simulink model "cx06_MA"  (Simulink 7.5)
settings: Solver=FixedStepDiscrete  StartTime=0.0  StopTime=10.0  RelTol=1e-3
undefined symbols (not defined in the file or in its folder): DiscIntNeverNeededParam, ECU555, int, motohawk_build_version, motohawk_trunc_name, motohawk_vardec_path
libraries: MotoHawk_lib x811, simulink x43, simulink_need_slupdate x1
(part 7 of 10)

== system cx06_MA/Strategy/Hybrid Control Code/Activation of Traction Control ==
  Inputs : Inport  OutDataType=sfix(16)  OutScaling=2^0
  Data1 : DataTypeConversion  OutDataTypeMode=uint8  OutDataType=sfix(16)  OutScaling=2^0  OutDataTypeStr=uint8
  Data2 : DataTypeConversion  OutDataTypeMode=uint8  OutDataType=sfix(16)  OutScaling=2^0  OutDataTypeStr=uint8
  Logical Operator : Logic  Operator=NOT  AllPortsSameDT=off  OutDataTypeMode=boolean  OutDataTypeStr=boolean
  Logical Operator1 : Logic  AllPortsSameDT=off  OutDataTypeMode=boolean  OutDataTypeStr=boolean
  Logical Operator2 : Logic  Operator=OR  AllPortsSameDT=off  OutDataTypeMode=boolean  OutDataTypeStr=boolean
  Logical Operator3 : Logic  Operator=OR  AllPortsSameDT=off  OutDataTypeMode=boolean  OutDataTypeStr=boolean
  Logical Operator4 : Logic  AllPortsSameDT=off  OutDataTypeMode=boolean  OutDataTypeStr=boolean
  Merge : Merge
  Merge1 : Merge  AllowUnequalInputPortWidths=on
  RRef_Wheel Diff : Subsystem  TreatAsAtomicUnit=on
  Switch Case : SwitchCase  CaseConditions={0,1}  ShowDefaultCase=off
  Wheel_Acceleration : Subsystem  TreatAsAtomicUnit=on
  motohawk_calibration : MotoHawk_lib/Calibration & Probing Blocks/motohawk_calibration  nam='Slip_Determine_Mode'  val=1  storage=Calibration  show_more=off  name_source=Use Parameter  data_type=Inherit from 'Default Value'  read_level=1  write_level=1  ovr_cals=on  view_as=Number  enum_struct={'Disabled', 'Enabled'}  vector_style=Wide Row  use_help_units=off  help=''  units=''  use_header_enum=off  row_header_enum={}  col_header_enum={}  use_min_max=off  min_val=-inf  max_val=inf  use_precision=off  precision=''  gain=1  offset=0  exp=1  use_mototune_group=off  mototune_group=motohawk_vardec_path(gcb)
  motohawk_data_def : MotoHawk_lib/Data Storage Blocks/motohawk_data_def  nam='inhibitTC'  container_nam=''  data=1  typ=uint8  struct_nam='MyStruct'  storage=NonVolatile  outputRef=off  use_vardec=on  window=Calibration  read_level=1  write_level=1  ovr_cals=on  view_as=Enumeration  enum_struct={'False','True'}  vector_style=Wide Row  use_help_units=on  help=''  units=''  use_header_enum=off  row_header_enum=''  col_header_enum=''  use_min_max=off  min_val=-inf  max_val=inf  use_precision=off  precision=''  gain=1  offset=0  exp=1  use_mototune_group=off  mototune_group=motohawk_vardec_path(gcb)  eval_name=inhibitTC  data_stores=motohawk_sfun_data_def_data_stores  struct_instances=motohawk_sfun_data_def_struct_instances  vardecs=motohawk_sfun_data_def_vardecs
  motohawk_data_def1 : MotoHawk_lib/Data Storage Blocks/motohawk_data_def  nam='TCVersion'  container_nam=''  data=1  typ=uint8  struct_nam='MyStruct'  storage=NonVolatile  outputRef=off  use_vardec=on  window=Calibration  read_level=1  write_level=1  ovr_cals=on  view_as=Enumeration  enum_struct={'Automatic','Manual'}  vector_style=Wide Row  use_help_units=on  help=''  units=''  use_header_enum=off  row_header_enum=''  col_header_enum=''  use_min_max=off  min_val=-inf  max_val=inf  use_precision=off  precision=''  gain=1  offset=0  exp=1  use_mototune_group=off  mototune_group=motohawk_vardec_path(gcb)  eval_name=TCVersion  data_stores=motohawk_sfun_data_def_data_stores  struct_instances=motohawk_sfun_data_def_struct_instances  vardecs=motohawk_sfun_data_def_vardecs
  motohawk_data_def2 : MotoHawk_lib/Data Storage Blocks/motohawk_data_def  nam='TC_Front_Slip'  container_nam=''  data=0  typ=uint8  struct_nam='MyStruct'  storage=Volatile  outputRef=off  use_vardec=off  window=Calibration  read_level=1  write_level=1  ovr_cals=on  view_as=Number  enum_struct={'Disabled', 'Enabled'}  vector_style=Wide Row  use_help_units=on  help=''  units=''  use_header_enum=off  row_header_enum=''  col_header_enum=''  use_min_max=off  min_val=-inf  max_val=inf  use_precision=off  precision=''  gain=1  offset=0  exp=1  use_mototune_group=off  mototune_group=motohawk_vardec_path(gcb)  eval_name=TC_Front_Slip  data_stores=motohawk_sfun_data_def_data_stores  struct_instances=motohawk_sfun_data_def_struct_instances  vardecs=motohawk_sfun_data_def_vardecs
  motohawk_data_def3 : MotoHawk_lib/Data Storage Blocks/motohawk_data_def  nam='TC_Rear_Slip'  container_nam=''  data=0  typ=uint8  struct_nam='MyStruct'  storage=Volatile  outputRef=off  use_vardec=off  window=Calibration  read_level=1  write_level=1  ovr_cals=on  view_as=Number  enum_struct={'Disabled', 'Enabled'}  vector_style=Wide Row  use_help_units=on  help=''  units=''  use_header_enum=off  row_header_enum=''  col_header_enum=''  use_min_max=off  min_val=-inf  max_val=inf  use_precision=off  precision=''  gain=1  offset=0  exp=1  use_mototune_group=off  mototune_group=motohawk_vardec_path(gcb)  eval_name=TC_Rear_Slip  data_stores=motohawk_sfun_data_def_data_stores  struct_instances=motohawk_sfun_data_def_struct_instances  vardecs=motohawk_sfun_data_def_vardecs
  motohawk_data_read : MotoHawk_lib/Data Storage Blocks/motohawk_data_read  source=Lookup By Name  structure=Scalar  operation=Read scalar from location by index  sz_vec=4  sz_row=2  sz_col=3  typ=uint8  nam='inhibitTC'  checkNull=on  struct_inst_name='Struct1'  struct_nam='MyStruct'
  motohawk_data_read1 : MotoHawk_lib/Data Storage Blocks/motohawk_data_read  source=Lookup By Name  structure=Scalar  operation=Read scalar from location by index  sz_vec=4  sz_row=2  sz_col=3  typ=uint8  nam='TCVersion'  checkNull=on  struct_inst_name='Struct1'  struct_nam='MyStruct'
  motohawk_data_write : MotoHawk_lib/Data Storage Blocks/motohawk_data_write  source=Lookup By Name  structure=Scalar  operation=Write scalar into location by index  sz_vec=-1  sz_row=3  sz_col=2  typ=uint8  nam='TC_Front_Slip'  checkNull=on  write_read_only=off  struct_inst_name='Struct1'  struct_name='MyStruct'
  motohawk_data_write1 : MotoHawk_lib/Data Storage Blocks/motohawk_data_write  source=Lookup By Name  structure=Scalar  operation=Write scalar into location by index  sz_vec=-1  sz_row=3  sz_col=2  typ=uint8  nam='TC_Rear_Slip'  checkNull=on  write_read_only=off  struct_inst_name='Struct1'  struct_name='MyStruct'
  motohawk_probe : MotoHawk_lib/Calibration & Probing Blocks/motohawk_probe  nam='Front_Slip'  show_more=on  name_source=Use Parameter  read_level=1  view_as=Number  enum_struct={'Disabled', 'Enabled'}  vector_style=Wide Row  use_help_units=off  help=''  units=''  use_header_enum=off  row_header_enum={}  col_header_enum={}  use_precision=off  precision=''  gain=1  offset=0  exp=1  use_mototune_group=off  mototune_group=motohawk_vardec_path(gcb)
  motohawk_probe1 : MotoHawk_lib/Calibration & Probing Blocks/motohawk_probe  nam='Rear_Slip'  show_more=on  name_source=Use Parameter  read_level=1  view_as=Number  enum_struct={'Disabled', 'Enabled'}  vector_style=Wide Row  use_help_units=off  help=''  units=''  use_header_enum=off  row_header_enum={}  col_header_enum={}  use_precision=off  precision=''  gain=1  offset=0  exp=1  use_mototune_group=off  mototune_group=motohawk_vardec_path(gcb)
  Front_Slip? : Outport  OutDataType=sfix(16)  OutScaling=2^0
  wires:
  motohawk_data_read/1 -> Logical Operator/1
  Logical Operator/1 -> Logical Operator1/1, Logical Operator4/1
  Logical Operator1/1 -> Front_Slip?/1, Data1/1
  motohawk_data_read1/1 -> Logical Operator3/1, Logical Operator2/1
  Logical Operator2/1 -> motohawk_probe/1, Logical Operator1/2  "Front_Slip?"
  Data1/1 -> motohawk_data_write/1
  Data2/1 -> motohawk_data_write1/1
  Logical Operator4/1 -> Data2/1
  Inputs/1 -> RRef_Wheel Diff/1(Inputs), Wheel_Acceleration/1(Inputs)
  Switch Case/1 -> RRef_Wheel Diff/Action
  Merge/1 -> Logical Operator2/2
  Merge1/1 -> Logical Operator3/2
  RRef_Wheel Diff/1(Front_Slip?) -> Merge/1
  RRef_Wheel Diff/2(Rear_Slip?) -> Merge1/1
  motohawk_calibration/1 -> Switch Case/1
  Switch Case/2 -> Wheel_Acceleration/Action
  Wheel_Acceleration/1(Front_Slip?) -> Merge/2
  Wheel_Acceleration/2(Rear_Slip?) -> Merge1/2
  Logical Operator3/1 -> motohawk_probe1/1, Logical Operator4/2

== system cx06_MA/Strategy/Hybrid Control Code/EBrake Disable ==
  Inputs : Inport  OutDataType=sfix(16)  OutScaling=2^0
  Sport Mode : Inport  Port=2  OutDataType=sfix(16)  OutScaling=2^0
  Bus Selector : BusSelector  OutputSignals=GMLAN.Park_Brake
  Constant : Constant  Value=-1  OutDataType=sfix(16)  OutScaling=2^0
  Constant1 : Constant  OutDataType=sfix(16)  OutScaling=2^0
  Gain : Gain  Gain=-1  ParameterDataType=sfix(16)  ParameterScaling=2^0  OutDataType=sfix(16)  OutScaling=2^0
  Logical Operator : Logic  AllPortsSameDT=off  OutDataTypeMode=Specify via dialog  OutDataTypeStr=uint(8)
  Product : Product  OutDataType=sfix(16)  OutScaling=2^0  RndMeth=Zero
  Relational Operator : RelationalOperator  Operator===  LogicOutDataTypeMode=boolean  OutDataTypeStr=boolean
  Saturation : Saturate  UpperLimit=1  LowerLimit=0
  Sum : Sum  Inputs=|++  OutDataType=sfix(16)  OutScaling=2^0
  motohawk_calibration : MotoHawk_lib/Calibration & Probing Blocks/motohawk_calibration  nam='Preload_Value'  val=.3  storage=Calibration  show_more=on  name_source=Use Parameter  data_type=double  read_level=1  write_level=1  ovr_cals=on  view_as=Number  enum_struct={'Disabled', 'Enabled'}  vector_style=Wide Row  use_help_units=off  help=''  units=''  use_header_enum=off  row_header_enum={}  col_header_enum={}  use_min_max=on  min_val=0  max_val=1  use_precision=on  precision='1.3'  gain=1  offset=0  exp=1  use_mototune_group=off  mototune_group=motohawk_vardec_path(gcb)
  Output : Outport  OutDataType=sfix(16)  OutScaling=2^0
  Offset : Outport  Port=2  OutDataType=sfix(16)  OutScaling=2^0
  wires:
  Inputs/1 -> Bus Selector/1
  Bus Selector/1 -> Sum/1, Relational Operator/2  "<Park_Brake>"
  Sum/1 -> Gain/1
  Saturation/1 -> Output/1
  Constant/1 -> Sum/2
  Constant1/1 -> Relational Operator/1
  Relational Operator/1 -> Logical Operator/1
  Sport Mode/1 -> Logical Operator/2
  Gain/1 -> Saturation/1
  Logical Operator/1 -> Product/1
  motohawk_calibration/1 -> Product/2
  Product/1 -> Offset/1

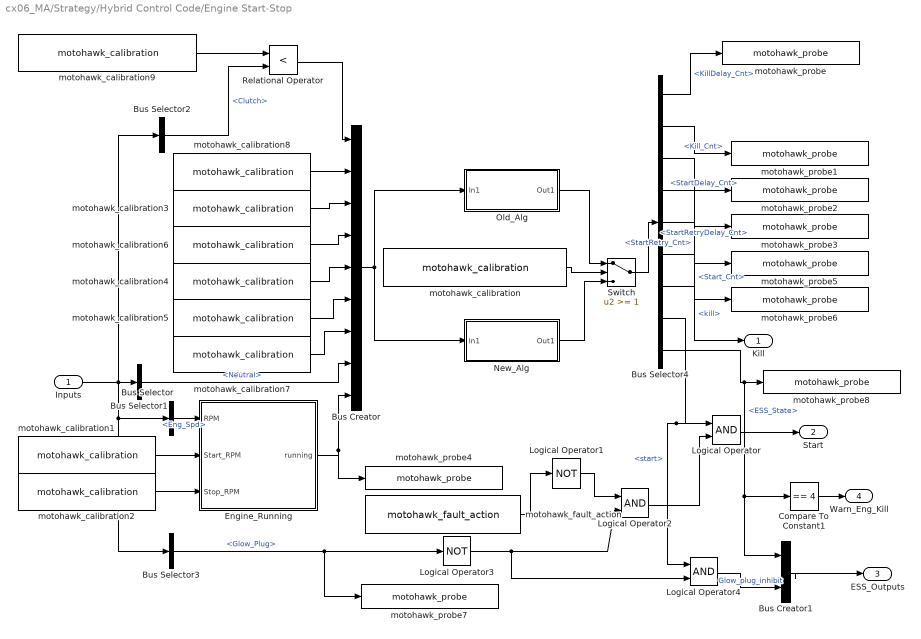
== system cx06_MA/Strategy/Hybrid Control Code/Engine Start-Stop ==
  Inputs : Inport  OutDataType=sfix(16)  OutScaling=2^0
  Bus Creator : BusCreator  Inputs=9
  Bus Creator1 : BusCreator  Inputs=2
  Bus Selector : BusSelector  OutputSignals=Fiat.Engine Speed and Pedal Pos.Eng_Spd
  Bus Selector1 : BusSelector  OutputSignals=Analog.Trans.Neutral
  Bus Selector2 : BusSelector  OutputSignals=Analog.Driver.Clutch
  Bus Selector3 : BusSelector  OutputSignals="Fiat.Engine  General Status.Glow_Plug"
  Bus Selector4 : BusSelector  OutputSignals=KillDelay_Cnt,Kill_Cnt,StartDelay_Cnt,StartRetryDelay_Cnt,StartRetry_Cnt,Start_Cnt,kill,start,ESS_State
  Compare To Constant1 : simulink/Logic and Bit Operations/Compare To Constant  SystemSampleTime=-1  relop===  const=4  LogicOutDataTypeMode=uint8  ZeroCross=off
  Engine_Running : Stateflow chart  TreatAsAtomicUnit=on
  Logical Operator : Logic  AllPortsSameDT=off  OutDataTypeMode=boolean  OutDataTypeStr=boolean
  Logical Operator1 : Logic  Operator=NOT  AllPortsSameDT=off  OutDataTypeMode=boolean  OutDataTypeStr=boolean
  Logical Operator2 : Logic  AllPortsSameDT=off  OutDataTypeMode=boolean  OutDataTypeStr=boolean
  Logical Operator3 : Logic  Operator=NOT  AllPortsSameDT=off  OutDataTypeMode=boolean  LogicDataType=fixdt(0, 8)  OutDataTypeStr=boolean
  Logical Operator4 : Logic  AllPortsSameDT=off  OutDataTypeMode=boolean  OutDataTypeStr=boolean
  New_Alg : Subsystem
  Old_Alg : Subsystem
  Relational Operator : RelationalOperator  Operator=<  LogicOutDataTypeMode=boolean  OutDataTypeStr=boolean
  Switch : Switch  Threshold=1
  motohawk_calibration : MotoHawk_lib/Calibration & Probing Blocks/motohawk_calibration  nam='EngineStopStartAlg'  val=1  storage=Calibration  show_more=on  name_source=Use Parameter  data_type=int8  read_level=1  write_level=1  ovr_cals=on  view_as=Enumeration  enum_struct={'ClutchControl', 'NeutralControl'}  vector_style=Wide Row  use_help_units=off  help=''  units=''  use_header_enum=off  row_header_enum={}  col_header_enum={}  use_min_max=off  min_val=-inf  max_val=inf  use_precision=off  precision=''  gain=1  offset=0  exp=1  use_mototune_group=off  mototune_group=motohawk_vardec_path(gcb)
  motohawk_calibration1 : MotoHawk_lib/Calibration & Probing Blocks/motohawk_calibration  nam='Engine_Start_RPM'  val=500  storage=Calibration  show_more=on  name_source=Use Parameter  data_type=Inherit from 'Default Value'  read_level=1  write_level=1  ovr_cals=on  view_as=Number  enum_struct={'Disabled', 'Enabled'}  vector_style=Wide Row  use_help_units=on  help='Engine is running above this speed'  units='rpm'  use_header_enum=off  row_header_enum={}  col_header_enum={}  use_min_max=off  min_val=-inf  max_val=inf  use_precision=off  precision=''  gain=1  offset=0  exp=1  use_mototune_group=off  mototune_group=motohawk_vardec_path(gcb)
  motohawk_calibration2 : MotoHawk_lib/Calibration & Probing Blocks/motohawk_calibration  nam='Engine_Stop_RPM'  val=50  storage=Calibration  show_more=on  name_source=Use Parameter  data_type=Inherit from 'Default Value'  read_level=1  write_level=1  ovr_cals=on  view_as=Number  enum_struct={'Disabled', 'Enabled'}  vector_style=Wide Row  use_help_units=on  help='Engine is not running below this speed'  units='rpm'  use_header_enum=off  row_header_enum={}  col_header_enum={}  use_min_max=off  min_val=-inf  max_val=inf  use_precision=off  precision=''  gain=1  offset=0  exp=1  use_mototune_group=off  mototune_group=motohawk_vardec_path(gcb)
  motohawk_calibration3 : MotoHawk_lib/Calibration & Probing Blocks/motohawk_calibration  nam='Kill_Time'  val=200  storage=Calibration  show_more=on  name_source=Use Parameter  data_type=uint16  read_level=1  write_level=1  ovr_cals=on  view_as=Number  enum_struct={'Disabled', 'Enabled'}  vector_style=Wide Row  use_help_units=on  help='Kill engine for this long'  units='s'  use_header_enum=off  row_header_enum={}  col_header_enum={}  use_min_max=off  min_val=0  max_val=50  use_precision=on  precision='1.1'  gain=0.005  offset=0  exp=1  use_mototune_group=off  mototune_group=motohawk_vardec_path(gcb)
  motohawk_calibration4 : MotoHawk_lib/Calibration & Probing Blocks/motohawk_calibration  nam='StartRetry_Delay'  val=400  storage=Calibration  show_more=on  name_source=Use Parameter  data_type=uint16  read_level=1  write_level=1  ovr_cals=on  view_as=Number  enum_struct={'Disabled', 'Enabled'}  vector_style=Wide Row  use_help_units=on  help='Try to start again this long after failing'  units='s'  use_header_enum=off  row_header_enum={}  col_header_enum={}  use_min_max=off  min_val=0  max_val=50  use_precision=on  precision='1.1'  gain=0.005  offset=0  exp=1  use_mototune_group=off  mototune_group=motohawk_vardec_path(gcb)
  motohawk_calibration5 : MotoHawk_lib/Calibration & Probing Blocks/motohawk_calibration  nam='Start_Delay'  val=40  storage=Calibration  show_more=on  name_source=Use Parameter  data_type=uint16  read_level=1  write_level=1  ovr_cals=on  view_as=Number  enum_struct={'Disabled', 'Enabled'}  vector_style=Wide Row  use_help_units=off  help='Must be out of neutral this long to start'  units='s'  use_header_enum=off  row_header_enum={}  col_header_enum={}  use_min_max=off  min_val=0  max_val=50  use_precision=on  precision='1.1'  gain=0.005  offset=0  exp=1  use_mototune_group=off  mototune_group=motohawk_vardec_path(gcb)
  motohawk_calibration6 : MotoHawk_lib/Calibration & Probing Blocks/motohawk_calibration  nam='Max_StartRetry'  val=4  storage=Calibration  show_more=on  name_source=Use Parameter  data_type=Inherit from 'Default Value'  read_level=1  write_level=1  ovr_cals=on  view_as=Number  enum_struct={'Disabled', 'Enabled'}  vector_style=Wide Row  use_help_units=on  help='After trying to start this many times, must put in neutral'  units=''  use_header_enum=off  row_header_enum={}  col_header_enum={}  use_min_max=off  min_val=-inf  max_val=inf  use_precision=off  precision=''  gain=1  offset=0  exp=1  use_mototune_group=off  mototune_group=motohawk_vardec_path(gcb)
  motohawk_calibration7 : MotoHawk_lib/Calibration & Probing Blocks/motohawk_calibration  nam='Start_Time'  val=400  storage=Calibration  show_more=on  name_source=Use Parameter  data_type=uint16  read_level=1  write_level=1  ovr_cals=on  view_as=Number  enum_struct={'Disabled', 'Enabled'}  vector_style=Wide Row  use_help_units=off  help='Max time to crank before failing'  units='s'  use_header_enum=off  row_header_enum={}  col_header_enum={}  use_min_max=on  min_val=0  max_val=50  use_precision=on  precision='1.1'  gain=0.005  offset=0  exp=1  use_mototune_group=off  mototune_group=motohawk_vardec_path(gcb)
  motohawk_calibration8 : MotoHawk_lib/Calibration & Probing Blocks/motohawk_calibration  nam='KillDelay'  val=1000  storage=Calibration  show_more=on  name_source=Use Parameter  data_type=uint16  read_level=1  write_level=1  ovr_cals=on  view_as=Number  enum_struct={'Disabled', 'Enabled'}  vector_style=Wide Row  use_help_units=off  help='Must be in neutral this long to kill'  units='s'  use_header_enum=off  row_header_enum={}  col_header_enum={}  use_min_max=on  min_val=0  max_val=50  use_precision=on  precision='1.1'  gain=0.005  offset=0  exp=1  use_mototune_group=off  mototune_group=motohawk_vardec_path(gcb)
  motohawk_calibration9 : MotoHawk_lib/Calibration & Probing Blocks/motohawk_calibration  nam='Clutch_Mech_Engage_in_ESS'  val=0.75  storage=Calibration  show_more=off  name_source=Use Parameter  data_type=Inherit from 'Default Value'  read_level=1  write_level=1  ovr_cals=on  view_as=Number  enum_struct={'Disabled', 'Enabled'}  vector_style=Wide Row  use_help_units=off  help=''  units=''  use_header_enum=off  row_header_enum={}  col_header_enum={}  use_min_max=off  min_val=-inf  max_val=inf  use_precision=off  precision=''  gain=1  offset=0  exp=1  use_mototune_group=off  mototune_group=motohawk_vardec_path(gcb)
  motohawk_fault_action : MotoHawk_lib/Fault Management Blocks/motohawk_fault_action  nam='inhibitEngineSS'  output_status=on  eval_nam=inhibitEngineSS
  motohawk_probe : MotoHawk_lib/Calibration & Probing Blocks/motohawk_probe  nam='KillDelay_Cnt'  show_more=on  name_source=Use Parameter  read_level=1  view_as=Number  enum_struct={'Disabled', 'Enabled'}  vector_style=Wide Row  use_help_units=off  help=''  units=''  use_header_enum=off  row_header_enum={}  col_header_enum={}  use_precision=on  precision=''  gain=0.005  offset=0  exp=1  use_mototune_group=off  mototune_group=motohawk_vardec_path(gcb)
  motohawk_probe1 : MotoHawk_lib/Calibration & Probing Blocks/motohawk_probe  nam='Kill_Cnt'  show_more=on  name_source=Use Parameter  read_level=1  view_as=Number  enum_struct={'Disabled', 'Enabled'}  vector_style=Wide Row  use_help_units=off  help=''  units=''  use_header_enum=off  row_header_enum={}  col_header_enum={}  use_precision=on  precision=''  gain=0.005  offset=0  exp=1  use_mototune_group=off  mototune_group=motohawk_vardec_path(gcb)
  motohawk_probe2 : MotoHawk_lib/Calibration & Probing Blocks/motohawk_probe  nam='StartDelay_Cnt'  show_more=on  name_source=Use Parameter  read_level=1  view_as=Number  enum_struct={'Disabled', 'Enabled'}  vector_style=Wide Row  use_help_units=off  help=''  units=''  use_header_enum=off  row_header_enum={}  col_header_enum={}  use_precision=on  precision=''  gain=0.005  offset=0  exp=1  use_mototune_group=off  mototune_group=motohawk_vardec_path(gcb)
  motohawk_probe3 : MotoHawk_lib/Calibration & Probing Blocks/motohawk_probe  nam='StartRetryDelay_Cnt'  show_more=on  name_source=Use Parameter  read_level=1  view_as=Number  enum_struct={'Disabled', 'Enabled'}  vector_style=Wide Row  use_help_units=off  help=''  units=''  use_header_enum=off  row_header_enum={}  col_header_enum={}  use_precision=on  precision=''  gain=.005  offset=0  exp=1  use_mototune_group=off  mototune_group=motohawk_vardec_path(gcb)
  motohawk_probe4 : MotoHawk_lib/Calibration & Probing Blocks/motohawk_probe  nam='Engine_Running'  show_more=on  name_source=Use Parameter  read_level=1  view_as=Enumeration  enum_struct={'False', 'True'}  vector_style=Wide Row  use_help_units=off  help=''  units=''  use_header_enum=off  row_header_enum={}  col_header_enum={}  use_precision=on  precision=''  gain=1  offset=0  exp=1  use_mototune_group=off  mototune_group=motohawk_vardec_path(gcb)
  motohawk_probe5 : MotoHawk_lib/Calibration & Probing Blocks/motohawk_probe  nam='StartRetry_Cnt'  show_more=off  name_source=Use Parameter  read_level=1  view_as=Number  enum_struct={'Disabled', 'Enabled'}  vector_style=Wide Row  use_help_units=off  help=''  units=''  use_header_enum=off  row_header_enum={}  col_header_enum={}  use_precision=off  precision=''  gain=1  offset=0  exp=1  use_mototune_group=off  mototune_group=motohawk_vardec_path(gcb)
  motohawk_probe6 : MotoHawk_lib/Calibration & Probing Blocks/motohawk_probe  nam='Start_Cnt'  show_more=on  name_source=Use Parameter  read_level=1  view_as=Number  enum_struct={'Disabled', 'Enabled'}  vector_style=Wide Row  use_help_units=off  help=''  units=''  use_header_enum=off  row_header_enum={}  col_header_enum={}  use_precision=on  precision=''  gain=0.005  offset=0  exp=1  use_mototune_group=off  mototune_group=motohawk_vardec_path(gcb)
  motohawk_probe7 : MotoHawk_lib/Calibration & Probing Blocks/motohawk_probe  nam='Eng_Glow_Plug_On'  show_more=on  name_source=Use Parameter  read_level=1  view_as=Number  enum_struct={'Disabled', 'Enabled'}  vector_style=Wide Row  use_help_units=off  help=''  units=''  use_header_enum=off  row_header_enum={}  col_header_enum={}  use_precision=on  precision=''  gain=1  offset=0  exp=1  use_mototune_group=off  mototune_group=motohawk_vardec_path(gcb)
  motohawk_probe8 : MotoHawk_lib/Calibration & Probing Blocks/motohawk_probe  nam='ESS_State'  show_more=on  name_source=Use Parameter  read_level=1  view_as=Enumeration  enum_struct={'Idle', 'StartDelay', 'Start', 'StartRetry', 'KillDelay', 'Kill', 'FalseStart'}  vector_style=Wide Row  use_help_units=off  help=''  units=''  use_header_enum=off  row_header_enum={}  col_header_enum={}  use_precision=on  precision=''  gain=1  offset=0  exp=1  use_mototune_group=off  mototune_group=motohawk_vardec_path(gcb)
  Kill : Outport  OutDataType=sfix(16)  OutScaling=2^0
  Start : Outport  Port=2  OutDataType=sfix(16)  OutScaling=2^0
  ESS_Outputs : Outport  Port=3  OutDataType=sfix(16)  OutScaling=2^0
  Warn_Eng_Kill : Outport  Port=4  OutDataType=sfix(16)  OutScaling=2^0
  wires:
  Logical Operator1/1 -> Logical Operator2/1
  Logical Operator2/1 -> Logical Operator/2
  Logical Operator/1 -> Start/1
  motohawk_fault_action/1 -> Logical Operator1/1
  Bus Selector2/1 -> Relational Operator/2  "<Clutch>"
  Engine_Running/1(running) -> motohawk_probe4/1, Bus Creator/9
  Bus Selector/1 -> Engine_Running/1(RPM)  "<Eng_Spd>"
  Inputs/1 -> Bus Selector2/1, Bus Selector1/1, Bus Selector3/1, Bus Selector/1
  motohawk_calibration2/1 -> Engine_Running/3(Stop_RPM)
  motohawk_calibration1/1 -> Engine_Running/2(Start_RPM)
  Relational Operator/1 -> Bus Creator/1
  motohawk_calibration8/1 -> Bus Creator/2
  motohawk_calibration3/1 -> Bus Creator/3
  motohawk_calibration6/1 -> Bus Creator/4
  motohawk_calibration4/1 -> Bus Creator/5
  motohawk_calibration5/1 -> Bus Creator/6
  motohawk_calibration7/1 -> Bus Creator/7
  Bus Selector1/1 -> Bus Creator/8  "<Neutral>"
  Bus Creator/1 -> New_Alg/1(In1), Old_Alg/1(In1)
  Old_Alg/1(Out1) -> Switch/1
  New_Alg/1(Out1) -> Switch/3
  motohawk_calibration/1 -> Switch/2
  Switch/1 -> Bus Selector4/1
  Bus Selector4/1 -> motohawk_probe/1  "<KillDelay_Cnt>"
  Bus Selector4/2 -> motohawk_probe1/1  "<Kill_Cnt>"
  Bus Selector4/3 -> motohawk_probe2/1  "<StartDelay_Cnt>"
  Bus Selector4/4 -> motohawk_probe3/1  "<StartRetryDelay_Cnt>"
  Bus Selector4/5 -> motohawk_probe5/1  "<StartRetry_Cnt>"
  Bus Selector4/6 -> motohawk_probe6/1  "<Start_Cnt>"
  Bus Selector4/7 -> Kill/1  "<kill>"
  Bus Selector4/8 -> Logical Operator/1, Logical Operator4/1  "<start>"
  Bus Selector4/9 -> motohawk_probe8/1, Bus Creator1/1, Compare To Constant1/1  "<ESS_State>"
  Bus Creator1/1 -> ESS_Outputs/1
  Logical Operator4/1 -> Bus Creator1/2  "Glow_plug_inhibit"
  Compare To Constant1/1 -> Warn_Eng_Kill/1
  Bus Selector3/1 -> motohawk_probe7/1, Logical Operator3/1  "<Glow_Plug>"
  Logical Operator3/1 -> Logical Operator4/2, Logical Operator2/2
  motohawk_calibration9/1 -> Relational Operator/1

== system cx06_MA/Strategy/Hybrid Control Code/HEV ==
  Inputs : Inport  OutDataType=sfix(16)  OutScaling=2^0
  RampInPt : Inport  Port=2  OutDataType=sfix(16)  OutScaling=2^0
  Activate_AT? : Inport  Port=3  OutDataType=sfix(16)  OutScaling=2^0
  Action Port : ActionPort  ActionType=case
  AssistedTakeOff : Subsystem
  Bus Creator : BusCreator  Inputs='engine_Torque','motor_Torque','motor_Enable'
  Bus Selector : BusSelector  OutputSignals=Analog.Driver.Accel
  Bus Selector1 : BusSelector  OutputSignals=Analog.Trans.Reverse,Analog.Driver.Accel
  Bus Selector2 : BusSelector  OutputSignals=JCI.SOC
  Constant : Constant  OutDataType=sfix(16)  OutScaling=2^0
  Constant1 : Constant  OutDataType=sfix(16)  OutScaling=2^0
  Constant2 : Constant  OutDataType=sfix(16)  OutScaling=2^0
  Data1 : DataTypeConversion  OutDataTypeMode=int8  OutDataType=sfix(16)  OutScaling=2^0  OutDataTypeStr=int8
  Divide : Product  Inputs=*/  OutDataType=sfix(16)  OutScaling=2^-10
  Gain : Gain  Gain=-2  ParameterDataType=sfix(16)  ParameterScaling=2^0  OutDataTypeMode=Specify via dialog  OutDataType=fixdt(1,8,0)  OutDataTypeStr=fixdt(1,8,0)
  Mult : Product  Inputs=**  OutDataType=sfix(16)  OutScaling=2^-10
  SOC_RampOut : Subsystem
  Saturation : Saturate  UpperLimit=1  LowerLimit=0
  Saturation1 : Saturate  UpperLimit=1  LowerLimit=-1
  Sum : Sum  Inputs=+-  OutDataType=sfix(16)  OutScaling=2^0
  Sum1 : Sum  Inputs=-+  OutDataType=sfix(16)  OutScaling=2^0
  Sum7 : Sum  Inputs=|++  OutDataType=sfix(16)  OutScaling=2^0
  motohawk_interpolation_1d_reference : MotoHawk_lib/Lookup Tables/motohawk_interpolation_1d_reference  nam='Diesel_Accel_MapTbl'  dt=double
  motohawk_prelookup_reference : MotoHawk_lib/Lookup Tables/motohawk_prelookup_reference  nam='Diesel_Accel_OrdIdxArr'  ref_nam=''  dt=double
  motohawk_probe2 : MotoHawk_lib/Calibration & Probing Blocks/motohawk_probe  nam='Dir_Component'  show_more=on  name_source=Use Parameter  read_level=1  view_as=Number  enum_struct={'False', 'True'}  vector_style=Wide Row  use_help_units=off  help=''  units=''  use_header_enum=off  row_header_enum={}  col_header_enum={}  use_precision=on  precision='1.3'  gain=1  offset=0  exp=1  use_mototune_group=off  mototune_group=motohawk_vardec_path(gcb)
  Outputs : Outport  OutDataType=sfix(16)  OutScaling=2^0  InitialOutput=0
  wires:
  motohawk_prelookup_reference/1 -> motohawk_interpolation_1d_reference/1
  Bus Creator/1 -> Outputs/1
  motohawk_interpolation_1d_reference/1 -> Bus Creator/1  "engine_Torque"
  Inputs/1 -> Bus Selector/1, Bus Selector1/1, Bus Selector2/1, AssistedTakeOff/2(Inputs)
  Bus Selector/1 -> motohawk_prelookup_reference/1  "<Accel>"
  RampInPt/1 -> Sum/2, Sum1/1
  Constant/1 -> Sum1/2
  Sum1/1 -> Divide/2
  Sum/1 -> Divide/1
  Divide/1 -> Saturation/1
  Constant1/1 -> Bus Creator/3  "motor_Enable"
  SOC_RampOut/1(Torque_Out) -> Saturation1/1
  Bus Selector2/1 -> SOC_RampOut/2(SOC)  "<SOC>"
  Activate_AT?/1 -> AssistedTakeOff/3(Activate?)
  Bus Selector1/1 -> Data1/1  "<Reverse>"
  Data1/1 -> Gain/1
  Constant2/1 -> Sum7/2
  Bus Selector1/2 -> Sum/1  "<Accel>"
  Gain/1 -> Sum7/1
  Saturation/1 -> AssistedTakeOff/1(T_in)
  Mult/1 -> SOC_RampOut/1(Torque_In)
  AssistedTakeOff/1(T_Out) -> Mult/2
  Sum7/1 -> Mult/1, motohawk_probe2/1
  Saturation1/1 -> Bus Creator/2  "motor_Torque"

== system cx06_MA/Strategy/Hybrid Control Code/Hybrid state limits ==
  note: Hybrid State
      | 0 - Safety
      | 1 - Diesel
      | 2 - Regen
      | 3 - HEV
      | 4 - ZEV
  state : Inport  OutDataType=sfix(16)  OutScaling=2^0
  Embedded MATLAB Function : Stateflow chart  TreatAsAtomicUnit=on
  Logical Operator{,1..2,5} (4 alike) : Logic  Operator=OR  AllPortsSameDT=off  OutDataTypeMode=boolean  OutDataTypeStr=boolean
  motohawk_calibration1 : MotoHawk_lib/Calibration & Probing Blocks/motohawk_calibration  nam='InhibitAssist'  val=0  storage=Calibration  show_more=on  name_source=Use Parameter  data_type=uint8  read_level=1  write_level=1  ovr_cals=on  view_as=Enumeration  enum_struct={'False', 'True'}  vector_style=Wide Row  use_help_units=off  help=''  units=''  use_header_enum=off  row_header_enum={}  col_header_enum={}  use_min_max=off  min_val=-inf  max_val=inf  use_precision=off  precision=''  gain=1  offset=0  exp=1  use_mototune_group=off  mototune_group=motohawk_vardec_path(gcb)
  motohawk_calibration3 : MotoHawk_lib/Calibration & Probing Blocks/motohawk_calibration  nam='InhibitZEV'  val=0  storage=Calibration  show_more=on  name_source=Use Parameter  data_type=uint8  read_level=1  write_level=1  ovr_cals=on  view_as=Enumeration  enum_struct={'False', 'True'}  vector_style=Wide Row  use_help_units=off  help=''  units=''  use_header_enum=off  row_header_enum={}  col_header_enum={}  use_min_max=off  min_val=-inf  max_val=inf  use_precision=off  precision=''  gain=1  offset=0  exp=1  use_mototune_group=off  mototune_group=motohawk_vardec_path(gcb)
  motohawk_data_def : MotoHawk_lib/Data Storage Blocks/motohawk_data_def  nam='inhibitRegen'  container_nam=''  data=0  typ=uint8  struct_nam='MyStruct'  storage=NonVolatile  outputRef=off  use_vardec=on  window=Calibration  read_level=1  write_level=1  ovr_cals=on  view_as=Enumeration  enum_struct={'False','True'}  vector_style=Wide Row  use_help_units=on  help=''  units=''  use_header_enum=off  row_header_enum=''  col_header_enum=''  use_min_max=off  min_val=-inf  max_val=inf  use_precision=off  precision=''  gain=1  offset=0  exp=1  use_mototune_group=off  mototune_group=motohawk_vardec_path(gcb)  eval_name=inhibitRegen  data_stores=motohawk_sfun_data_def_data_stores  struct_instances=motohawk_sfun_data_def_struct_instances  vardecs=motohawk_sfun_data_def_vardecs
  motohawk_data_read : MotoHawk_lib/Data Storage Blocks/motohawk_data_read  source=Lookup By Name  structure=Scalar  operation=Read scalar from location by index  sz_vec=4  sz_row=2  sz_col=3  typ=uint8  nam='inhibitRegen'  checkNull=on  struct_inst_name='Struct1'  struct_nam='MyStruct'
  motohawk_fault_action : MotoHawk_lib/Fault Management Blocks/motohawk_fault_action  nam='inhibitEV'  output_status=on  eval_nam=inhibitEV
  motohawk_fault_action1 : MotoHawk_lib/Fault Management Blocks/motohawk_fault_action  nam='inhibitRegen'  output_status=on  eval_nam=inhibitRegen
  motohawk_fault_action2 : MotoHawk_lib/Fault Management Blocks/motohawk_fault_action  nam='inhibitDiesel'  output_status=on  eval_nam=inhibitDiesel
  state_o : Outport  OutDataType=sfix(16)  OutScaling=2^0
  wires:
  Logical Operator1/1 -> Embedded MATLAB Function/4(nZEV)
  state/1 -> Embedded MATLAB Function/1(state)
  Embedded MATLAB Function/1(nState) -> state_o/1
  motohawk_fault_action2/1 -> Embedded MATLAB Function/2(nDiesel), Logical Operator5/1
  motohawk_calibration1/1 -> Logical Operator/1
  motohawk_fault_action/1 -> Logical Operator/2
  Logical Operator5/1 -> Embedded MATLAB Function/3(nHEV)
  Logical Operator/1 -> Logical Operator5/2, Logical Operator1/1
  motohawk_calibration3/1 -> Logical Operator1/2
  motohawk_fault_action1/1 -> Logical Operator2/2
  Logical Operator2/1 -> Embedded MATLAB Function/5(nRegen)
  motohawk_data_read/1 -> Logical Operator2/1

== system cx06_MA/Strategy/Hybrid Control Code/Ramp_In_Pt ==
  TC_Front_Slip? : Inport  OutDataType=sfix(16)  OutScaling=2^0
  Inputs : Inport  Port=2  OutDataType=sfix(16)  OutScaling=2^0
  Bus Selector : BusSelector  OutputSignals=Analog.Driver.Accel
  Bus Selector1 : BusSelector  OutputSignals=JCI.SOC
  Constant : Constant  OutDataType=sfix(16)  OutScaling=2^0
  Constant1 : Constant  OutDataType=sfix(16)  OutScaling=2^0
  Gain : Gain  Gain=1/100  ParameterDataType=sfix(16)  ParameterScaling=2^0  OutDataType=sfix(16)  OutScaling=2^0
  Gain1 : Gain  Gain=-1/200  ParameterDataType=sfix(16)  ParameterScaling=2^0  OutDataType=sfix(16)  OutScaling=2^0
  Gain2 : Gain  Gain=-1  ParameterDataType=sfix(16)  ParameterScaling=2^0  OutDataType=sfix(16)  OutScaling=2^0
  Math Function1 : Math  Operator=reciprocal  OutDataType=sfix(16)  OutScaling=2^0  SaturateOnIntegerOverflow=on
  MinMax : MinMax  Inputs=2  OutDataType=sfix(16)  OutScaling=2^0
  Product : Product  OutDataType=sfix(16)  OutScaling=2^0  RndMeth=Zero
  Product1 : Product  OutDataType=sfix(16)  OutScaling=2^0  RndMeth=Zero
  Saturation : Saturate  UpperLimit=0.8  LowerLimit=0
  Saturation1 : Saturate  UpperLimit=1  LowerLimit=0
  Saturation2 : Saturate  UpperLimit=1  LowerLimit=0
  Sum : Sum  Inputs=|++  OutDataType=sfix(16)  OutScaling=2^0
  Sum1 : Sum  Inputs=|-+  OutDataType=sfix(16)  OutScaling=2^0
  Sum2 : Sum  OutDataType=sfix(16)  OutScaling=2^0
  Sum3 : Sum  Inputs=++|  OutDataType=sfix(16)  OutScaling=2^0
  Switch : Switch  Criteria=u2 > Threshold
  Switch2 : Switch  Threshold=1
  Switch6 : Switch  Criteria=u2 > Threshold
  Unit Delay1 : UnitDelay  SampleTime=-1
  Unit Delay2 : UnitDelay  X0=1  SampleTime=-1
  motohawk_calibration1 : MotoHawk_lib/Calibration & Probing Blocks/motohawk_calibration  nam='Filt_Accel_K'  val=.0005  storage=Calibration  show_more=on  name_source=Use Parameter  data_type=Inherit from 'Default Value'  read_level=1  write_level=1  ovr_cals=on  view_as=Number  enum_struct={'Disabled', 'Enabled'}  vector_style=Wide Row  use_help_units=off  help='new*K+old*(1-K)'  units=''  use_header_enum=off  row_header_enum={}  col_header_enum={}  use_min_max=off  min_val=0  max_val=1  use_precision=on  precision='1.4'  gain=1  offset=0  exp=1  use_mototune_group=off  mototune_group=motohawk_vardec_path(gcb)
  motohawk_calibration3 : MotoHawk_lib/Calibration & Probing Blocks/motohawk_calibration  nam='TC_Rmp_Adjust_Rate'  val=2  storage=Calibration  show_more=on  name_source=Use Parameter  data_type=Inherit from 'Default Value'  read_level=1  write_level=1  ovr_cals=on  view_as=Number  enum_struct={'Disabled', 'Enabled'}  vector_style=Wide Row  use_help_units=on  help='time it takes to ramp down max torque available from 1 to 0'  units='sec'  use_header_enum=off  row_header_enum={}  col_header_enum={}  use_min_max=on  min_val=0.001  max_val=inf  use_precision=on  precision='1.4'  gain=1  offset=0  exp=1  use_mototune_group=off  mototune_group=motohawk_vardec_path(gcb)
  motohawk_interpolation_1d : MotoHawk_lib/Lookup Tables/motohawk_interpolation_1d  nam='RampInPt_SOC'  table_data=[50:-5:10]  show_more=off  data_type=Inherit from 'Table Data'  storage=NonAdaptive  read_level=1  write_level=1  ovr_cals=on  use_help=off  help=''  units=''  use_min_max=off  min_val=-inf  max_val=inf  use_precision=off  precision=''  gain=1  offset=0  exp=1  use_links=off  prelookup_block=''  output_name=''  use_mototune_group=off  mototune_group=motohawk_vardec_path(gcb)
  motohawk_prelookup : MotoHawk_lib/Lookup Tables/motohawk_prelookup  nam='RampInPt_SOC_Ord'  breakpoint_data=[10:5:50]  show_more=on  data_type=Inherit from 'Table Data'  storage=NonVolatile  read_level=1  write_level=1  ovr_cals=on  use_help=off  help=''  units='%'  use_min_max=off  min_val=-inf  max_val=inf  use_precision=off  precision=''  gain=1  offset=0  exp=1  use_links=off  input_name=''  use_mototune_group=off  mototune_group=motohawk_vardec_path(gcb)
  motohawk_probe : MotoHawk_lib/Calibration & Probing Blocks/motohawk_probe  nam='Filt_Accel'  show_more=off  name_source=Use Parameter  read_level=1  view_as=Number  enum_struct={'Disabled', 'Enabled'}  vector_style=Wide Row  use_help_units=off  help=''  units=''  use_header_enum=off  row_header_enum={}  col_header_enum={}  use_precision=off  precision=''  gain=1  offset=0  exp=1  use_mototune_group=off  mototune_group=motohawk_vardec_path(gcb)
  motohawk_probe1 : MotoHawk_lib/Calibration & Probing Blocks/motohawk_probe  nam='Ramp_In_Pt'  show_more=off  name_source=Use Parameter  read_level=1  view_as=Number  enum_struct={'Disabled', 'Enabled'}  vector_style=Wide Row  use_help_units=off  help=''  units=''  use_header_enum=off  row_header_enum={}  col_header_enum={}  use_precision=off  precision=''  gain=1  offset=0  exp=1  use_mototune_group=off  mototune_group=motohawk_vardec_path(gcb)
  motohawk_probe2 : MotoHawk_lib/Calibration & Probing Blocks/motohawk_probe  nam='SOC_Component'  show_more=off  name_source=Use Parameter  read_level=1  view_as=Number  enum_struct={'Disabled', 'Enabled'}  vector_style=Wide Row  use_help_units=off  help=''  units=''  use_header_enum=off  row_header_enum={}  col_header_enum={}  use_precision=off  precision=''  gain=1  offset=0  exp=1  use_mototune_group=off  mototune_group=motohawk_vardec_path(gcb)
  motohawk_probe3 : MotoHawk_lib/Calibration & Probing Blocks/motohawk_probe  nam='Pedal_Component'  show_more=off  name_source=Use Parameter  read_level=1  view_as=Number  enum_struct={'Disabled', 'Enabled'}  vector_style=Wide Row  use_help_units=off  help=''  units=''  use_header_enum=off  row_header_enum={}  col_header_enum={}  use_precision=off  precision=''  gain=1  offset=0  exp=1  use_mototune_group=off  mototune_group=motohawk_vardec_path(gcb)
  motohawk_probe4 : MotoHawk_lib/Calibration & Probing Blocks/motohawk_probe  nam='TC_Floater'  show_more=off  name_source=Use Parameter  read_level=1  view_as=Number  enum_struct={'Disabled', 'Enabled'}  vector_style=Wide Row  use_help_units=off  help=''  units=''  use_header_enum=off  row_header_enum={}  col_header_enum={}  use_precision=off  precision=''  gain=1  offset=0  exp=1  use_mototune_group=off  mototune_group=motohawk_vardec_path(gcb)
  rampInPt : Outport  OutDataType=sfix(16)  OutScaling=2^0
  wires:
  Inputs/1 -> Bus Selector/1, Bus Selector1/1
  Bus Selector/1 -> Product/1  "<Accel>"
  motohawk_calibration1/1 -> Product/2, Sum1/1
  Product/1 -> Sum/1
  Constant/1 -> Sum1/2
  Sum1/1 -> Product1/1
  Product1/1 -> Sum/2
  Unit Delay1/1 -> Product1/2
  Sum/1 -> motohawk_probe/1, Unit Delay1/1, Saturation1/1
  Bus Selector1/1 -> motohawk_prelookup/1  "<SOC>"
  motohawk_prelookup/1 -> motohawk_interpolation_1d/1
  Sum2/1 -> Saturation/1
  Saturation/1 -> rampInPt/1, motohawk_probe1/1
  motohawk_interpolation_1d/1 -> Gain/1
  Gain/1 -> Sum2/1, motohawk_probe2/1
  Unit Delay2/1 -> Sum3/2, Switch2/2
  Switch/1 -> Sum3/1
  motohawk_calibration3/1 -> Math Function1/1
  Gain1/1 -> Switch/1, Gain2/1
  Sum3/1 -> Switch2/3
  Math Function1/1 -> Gain1/1
  TC_Front_Slip?/1 -> Switch/2, Switch6/2  "Front_Slip?"
  Switch6/1 -> Switch2/1
  Constant1/1 -> Switch6/3
  Switch2/1 -> Saturation2/1, motohawk_probe4/1
  Gain2/1 -> Switch/3
  Saturation1/1 -> Switch6/1, MinMax/1
  MinMax/1 -> Sum2/2, motohawk_probe3/1
  Saturation2/1 -> Unit Delay2/1, MinMax/2

== system cx06_MA/Strategy/Hybrid Control Code/Regen ==
  Inputs : Inport  OutDataType=sfix(16)  OutScaling=2^0
  Action Port : ActionPort  ActionType=case
  Bus Creator : BusCreator  Inputs='engine_Torque','motor_Torque','motor_Enable'
  Bus Selector : BusSelector  OutputSignals=Analog.Driver.Accel
  Bus Selector1 : BusSelector  OutputSignals=Analog.Driver.Brake
  Bus Selector2 : BusSelector  OutputSignals=IPT.Status 2.veh_speed,JCI.SOC
  Constant1 : Constant  OutDataType=sfix(16)  OutScaling=2^0
  Divide : Product  Inputs=*/  OutDataType=sfix(16)  OutScaling=2^-10
  Gain : Gain  Gain=-1  ParameterDataType=sfix(16)  ParameterScaling=2^0  OutDataType=sfix(16)  OutScaling=2^0
  SOC_RampOut : Subsystem
  Saturation : Saturate  UpperLimit=0  LowerLimit=-1
  Sum : Sum  Inputs=+-  OutDataType=sfix(16)  OutScaling=2^0
  Sum1 : Sum  Inputs=-+  OutDataType=sfix(16)  OutScaling=2^0
  motohawk_calibration2 : MotoHawk_lib/Calibration & Probing Blocks/motohawk_calibration  nam='Regen_Full'  val=.3  storage=Calibration  show_more=on  name_source=Use Parameter  data_type=Inherit from 'Default Value'  read_level=1  write_level=1  ovr_cals=on  view_as=Number  enum_struct={'Disabled', 'Enabled'}  vector_style=Wide Row  use_help_units=off  help='Pedal Position where regen is Full'  units='%'  use_header_enum=off  row_header_enum={}  col_header_enum={}  use_min_max=on  min_val=0  max_val=2  use_precision=off  precision='1.2'  gain=1  offset=0  exp=1  use_mototune_group=off  mototune_group=motohawk_vardec_path(gcb)
  motohawk_data_def2 : MotoHawk_lib/Data Storage Blocks/motohawk_data_def  nam='Regen_Start'  container_nam=''  data=.03  typ=double  struct_nam='MyStruct'  storage=NonVolatile  outputRef=off  use_vardec=on  window=Calibration  read_level=1  write_level=1  ovr_cals=on  view_as=Number  enum_struct={'Disabled', 'Enabled'}  vector_style=Wide Row  use_help_units=off  help='Regen Starts above this position'  units='%'  use_header_enum=off  row_header_enum=''  col_header_enum=''  use_min_max=off  min_val=0  max_val=1  use_precision=off  precision='1.2'  gain=1  offset=0  exp=1  use_mototune_group=off  mototune_group=motohawk_vardec_path(gcb)  eval_name=Regen_Start  data_stores=motohawk_sfun_data_def_data_stores  struct_instances=motohawk_sfun_data_def_struct_instances  vardecs=motohawk_sfun_data_def_vardecs
  motohawk_data_read1 : MotoHawk_lib/Data Storage Blocks/motohawk_data_read  source=Lookup By Name  structure=Scalar  operation=Read scalar from location by index  sz_vec=4  sz_row=2  sz_col=3  typ=double  nam='Regen_Start'  checkNull=on  struct_inst_name='Struct1'  struct_nam='MyStruct'
  motohawk_interpolation_1d_reference : MotoHawk_lib/Lookup Tables/motohawk_interpolation_1d_reference  nam='Diesel_Accel_MapTbl'  dt=double
  motohawk_prelookup_reference : MotoHawk_lib/Lookup Tables/motohawk_prelookup_reference  nam='Diesel_Accel_OrdIdxArr'  ref_nam=''  dt=double
  motohawk_probe : MotoHawk_lib/Calibration & Probing Blocks/motohawk_probe  nam='after_saturation'  show_more=on  name_source=Use Parameter  read_level=1  view_as=Number  enum_struct={'Disabled', 'Enabled'}  vector_style=Wide Row  use_help_units=off  help=''  units=''  use_header_enum=off  row_header_enum={}  col_header_enum={}  use_precision=on  precision='1.2'  gain=1  offset=0  exp=1  use_mototune_group=off  mototune_group=motohawk_vardec_path(gcb)
  motohawk_probe1 : MotoHawk_lib/Calibration & Probing Blocks/motohawk_probe  nam='speed_ramp_out'  show_more=on  name_source=Use Parameter  read_level=1  view_as=Number  enum_struct={'Disabled', 'Enabled'}  vector_style=Wide Row  use_help_units=off  help=''  units=''  use_header_enum=off  row_header_enum={}  col_header_enum={}  use_precision=on  precision='1.2'  gain=1  offset=0  exp=1  use_mototune_group=off  mototune_group=motohawk_vardec_path(gcb)
  speed_RampOut : Subsystem
  Outputs : Outport  OutDataType=sfix(16)  OutScaling=2^0  InitialOutput=0
  wires:
  Constant1/1 -> Bus Creator/3  "motor_Enable"
  motohawk_prelookup_reference/1 -> motohawk_interpolation_1d_reference/1
  Bus Creator/1 -> Outputs/1
  motohawk_interpolation_1d_reference/1 -> Bus Creator/1  "engine_Torque"
  Inputs/1 -> Bus Selector/1, Bus Selector1/1, Bus Selector2/1
  Bus Selector/1 -> motohawk_prelookup_reference/1  "<Accel>"
  Bus Selector1/1 -> Sum/1  "<Brake>"
  motohawk_data_read1/1 -> Sum/2, Sum1/1
  motohawk_calibration2/1 -> Sum1/2
  Sum/1 -> Divide/1
  Sum1/1 -> Divide/2
  Divide/1 -> Gain/1
  Gain/1 -> Saturation/1
  Saturation/1 -> speed_RampOut/1(Torque_In), motohawk_probe/1  "motor_Torque"
  speed_RampOut/1(Torque_Out) -> SOC_RampOut/1(Torque_In), motohawk_probe1/1
  SOC_RampOut/1(Torque_Out) -> Bus Creator/2  "motor_Torque"
  Bus Selector2/2 -> SOC_RampOut/2(SOC)  "<SOC>"
  Bus Selector2/1 -> speed_RampOut/2(speed)  "<veh_speed>"

== system cx06_MA/Strategy/Hybrid Control Code/Rev_Limiter ==
  Inputs : Inport  OutDataType=sfix(16)  OutScaling=2^0
  Torq_In : Inport  Port=2  OutDataType=sfix(16)  OutScaling=2^0
  Bus Selector : BusSelector  OutputSignals=IPT.Status 2.veh_speed,Analog.Driver.Clutch
  MinMax : MinMax  Inputs=2  OutDataType=sfix(16)  OutScaling=2^0
  Relational Operator : RelationalOperator  Operator=>  LogicOutDataTypeMode=Specify via dialog  OutDataTypeStr=uint(8)
  Relational Operator1 : RelationalOperator  Operator=<  LogicOutDataTypeMode=Specify via dialog  OutDataTypeStr=uint(8)
  Switch : Switch  Threshold=1
  Switch1 : Switch  Threshold=1
  Switch2 : Switch  Threshold=1
  motohawk_calibration : MotoHawk_lib/Calibration & Probing Blocks/motohawk_calibration  nam='Clutch_Thres_Shifts'  val=.6  storage=Calibration  show_more=on  name_source=Use Parameter  data_type=Inherit from 'Default Value'  read_level=1  write_level=1  ovr_cals=on  view_as=Number  enum_struct={'Disabled', 'Enabled'}  vector_style=Wide Row  use_help_units=off  help=''  units=''  use_header_enum=off  row_header_enum={}  col_header_enum={}  use_min_max=on  min_val=0  max_val=1.1  use_precision=on  precision='1.2'  gain=1  offset=0  exp=1  use_mototune_group=off  mototune_group=motohawk_vardec_path(gcb)
  motohawk_calibration1 : MotoHawk_lib/Calibration & Probing Blocks/motohawk_calibration  nam='Eng_Torq_Shifts'  val=.23  storage=Calibration  show_more=on  name_source=Use Parameter  data_type=Inherit from 'Default Value'  read_level=1  write_level=1  ovr_cals=on  view_as=Number  enum_struct={'Disabled', 'Enabled'}  vector_style=Wide Row  use_help_units=off  help=''  units=''  use_header_enum=off  row_header_enum={}  col_header_enum={}  use_min_max=on  min_val=0  max_val=1.1  use_precision=on  precision='1.3'  gain=1  offset=0  exp=1  use_mototune_group=off  mototune_group=motohawk_vardec_path(gcb)
  motohawk_calibration2 : MotoHawk_lib/Calibration & Probing Blocks/motohawk_calibration  nam='Eng_Torq_Take_Off'  val=.230  storage=Calibration  show_more=on  name_source=Use Parameter  data_type=Inherit from 'Default Value'  read_level=1  write_level=1  ovr_cals=on  view_as=Number  enum_struct={'Disabled', 'Enabled'}  vector_style=Wide Row  use_help_units=off  help=''  units=''  use_header_enum=off  row_header_enum={}  col_header_enum={}  use_min_max=on  min_val=0  max_val=1.1  use_precision=on  precision='1.3'  gain=1  offset=0  exp=1  use_mototune_group=off  mototune_group=motohawk_vardec_path(gcb)
  motohawk_calibration3 : MotoHawk_lib/Calibration & Probing Blocks/motohawk_calibration  nam='Speed_Threshold'  val=5  storage=Calibration  show_more=on  name_source=Use Parameter  data_type=Inherit from 'Default Value'  read_level=1  write_level=1  ovr_cals=on  view_as=Number  enum_struct={'Disabled', 'Enabled'}  vector_style=Wide Row  use_help_units=on  help=''  units='mph'  use_header_enum=off  row_header_enum={}  col_header_enum={}  use_min_max=on  min_val=0  max_val=60  use_precision=on  precision='1'  gain=1  offset=0  exp=1  use_mototune_group=off  mototune_group=motohawk_vardec_path(gcb)
  motohawk_calibration4 : MotoHawk_lib/Calibration & Probing Blocks/motohawk_calibration  nam='Clutch_Thres_Take_Off'  val=.76  storage=Calibration  show_more=on  name_source=Use Parameter  data_type=Inherit from 'Default Value'  read_level=1  write_level=1  ovr_cals=on  view_as=Number  enum_struct={'Disabled', 'Enabled'}  vector_style=Wide Row  use_help_units=off  help=''  units=''  use_header_enum=off  row_header_enum={}  col_header_enum={}  use_min_max=on  min_val=0  max_val=1.1  use_precision=on  precision='1.2'  gain=1  offset=0  exp=1  use_mototune_group=off  mototune_group=motohawk_vardec_path(gcb)
  Torq_Out : Outport  OutDataType=sfix(16)  OutScaling=2^0
  wires:
  Inputs/1 -> Bus Selector/1
  Bus Selector/2 -> Relational Operator/1  "<Clutch>"
  Relational Operator/1 -> Switch/2
  MinMax/1 -> Switch/1
  Switch/1 -> Torq_Out/1
  Switch1/1 -> MinMax/1
  Bus Selector/1 -> Relational Operator1/2  "<veh_speed>"
  Relational Operator1/1 -> Switch1/2, Switch2/2
  motohawk_calibration3/1 -> Relational Operator1/1
  motohawk_calibration1/1 -> Switch1/1
  motohawk_calibration2/1 -> Switch1/3
  Torq_In/1 -> Switch/3, MinMax/2
  Switch2/1 -> Relational Operator/2
  motohawk_calibration/1 -> Switch2/1
  motohawk_calibration4/1 -> Switch2/3

== system cx06_MA/Strategy/Hybrid Control Code/Safety ==
  Inputs : Inport  OutDataType=sfix(16)  OutScaling=2^0
  Action Port : ActionPort  ActionType=case
  Bus Creator : BusCreator  Inputs=3
  Constant : Constant  Value=0  OutDataType=sfix(16)  OutScaling=2^0
  Constant1 : Constant  Value=0  OutDataType=sfix(16)  OutScaling=2^0
  Constant2 : Constant  Value=0  OutDataType=sfix(16)  OutScaling=2^0
  Terminator : Terminator
  Outputs : Outport  OutDataType=sfix(16)  OutScaling=2^0  InitialOutput=0
  wires:
  Bus Creator/1 -> Outputs/1
  Constant/1 -> Bus Creator/2  "motor_Torque"
  Constant1/1 -> Bus Creator/1  "engine_Torque"
  Constant2/1 -> Bus Creator/3  "motor_Enable"
  Inputs/1 -> Terminator/1
